simulink model "chart_input"  (Simulink 6.3)
settings: Solver=ode45  StartTime=0.0  StopTime=10.0  RelTol=1e-3
settings Model: LastModifiedBy=deissenb

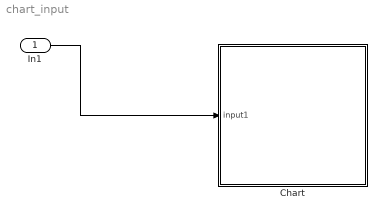
== system chart_input ==
  In1 : Inport
  Chart : Stateflow chart
  wires:
  In1/1 -> Chart/1(input1)

== stateflow chart Chart ==
  data: input1 input inherited
